simulink model "target_transmit"  (R2018a)
settings: Solver=FixedStepDiscrete  StartTime=0  StopTime=inf  RelTol=1e-3  EnableMultiTasking=on
InitFcn:
  | load data/bestsimulink_data
  | load data/bestsimulink320x240_data
  | load busObjects
StopFcn:
  | clear bestsimulink320x240_data
  | clear bestsimulink_data
  | clear dataBusObject
model workspace (MAT data in the model file):
  dt = 0.1
undefined symbols (not defined in the file or in its folder): gray, IsPositionTracked, IsSkeletonTracked, JointDepthIndices, JointImageIndices, JointTrackingState, JointWorldCoordinates, none, PositionDepthIndices, PositionImageIndices, PositionWorldCoordinates, Rec, SDTV, SegmentationData, SkeletonTrackingID, videoinput
libraries: visiontextngfix x24, embdlinuxlib x13, visionstatistics x7, visionconversions x5, visiontransforms x3, visionsinks x2, visionanalysis x1, dspvision x1, imaqlib x1, sldrtlib x1
(part 2 of 2)

== system target_transmit/Draw Bounding Boxes/No Comparison/Insert Buoy Blobs1 ==
  Video In : Inport
  Blob Data : Inport  Port=2
  Bus Selector : BusSelector  OutputSignals=green_bbox,red_bbox
  Draw Shapes Green : visiontextngfix/Draw Shapes  shape=Rectangles  fill=on  lineWidth=1  fillClrSource=Specify via dialog  display=User-specified value  intensity=200  color=[0 255 0]  opacity=0.6  viewport=Entire image  antialiasing=off  inType=Obsolete  imagePorts=One multidimensional signal  prodOutputMode=Binary point scaling  prodOutputWordLength=32  prodOutputFracLength=14  memoryMode=Specify word length  memoryWordLength=16  memoryFracLength=14  roundingMode=Floor  overflowMode=off
      settings: SourceProductName=Computer Vision System Toolbox
  Draw Shapes Red : visiontextngfix/Draw Shapes  shape=Rectangles  fill=on  lineWidth=1  fillClrSource=Specify via dialog  display=User-specified value  intensity=200  color=[255 0 0]  opacity=0.6  viewport=Entire image  antialiasing=off  inType=Obsolete  imagePorts=One multidimensional signal  prodOutputMode=Binary point scaling  prodOutputWordLength=32  prodOutputFracLength=14  memoryMode=Specify word length  memoryWordLength=16  memoryFracLength=14  roundingMode=Floor  overflowMode=off
      settings: SourceProductName=Computer Vision System Toolbox
  Video Out : Outport
  wires:
  Blob Data/1 -> Bus Selector/1
  Video In/1 -> Draw Shapes Green/1
  Draw Shapes Green/1 -> Draw Shapes Red/1
  Draw Shapes Red/1 -> Video Out/1
  Bus Selector/1 -> Draw Shapes Green/2  "<green_bbox>"
  Bus Selector/2 -> Draw Shapes Red/2  "<red_bbox>"

== system target_transmit/Draw Bounding Boxes/No Comparison/Insert Closest Text ==
  Video In : Inport
  Blob Data : Inport  Port=2
  Bus Selector : BusSelector  OutputSignals=green_area,green_centroid,green_bbox,red_area,red_centroid,red_bbox
  Convert Bus to Double : Subsystem  Commented=on
  Find Closest Buoy : MATLAB Function  TreatAsAtomicUnit=on
  Insert Text Green Closest : visiontextngfix/Insert Text  inputType=Obsolete  theText='Closest Green Buoy'  getTextLocFrom=Input port  textLoc=[1 1]  getTextColorFrom=Specify via dialog  textColor=[0 255 0]  getTextIntensityFrom=Specify via dialog  textIntensity=0  getTextOpacityFrom=Specify via dialog  textOpacity=1.0  dummyVar2=0  dummyVar3=0  dummyVar4=0  imagePorts=One multidimensional signal  isInputTransposed=off  fontFace=LucidaSansRegular  dummyVar1=0  blockFontSize=12  antiAliased=on
      settings: SourceProductName=Computer Vision System Toolbox  SourceProductBaseCode=VP
  Insert Text Red Closest : visiontextngfix/Insert Text  inputType=Obsolete  theText='Closest Red Buoy'  getTextLocFrom=Input port  textLoc=[1 1]  getTextColorFrom=Specify via dialog  textColor=[255 0 0]  getTextIntensityFrom=Specify via dialog  textIntensity=0  getTextOpacityFrom=Specify via dialog  textOpacity=1.0  dummyVar2=0  dummyVar3=0  dummyVar4=0  imagePorts=One multidimensional signal  isInputTransposed=off  fontFace=LucidaSansRegular  dummyVar1=0  blockFontSize=12  antiAliased=on
      settings: SourceProductName=Computer Vision System Toolbox  SourceProductBaseCode=VP
  To Workspace : ToWorkspace  Commented=on  VariableName=data1  SaveFormat=Timeseries  SampleTime=-1
  Video Out : Outport
  wires:
  Insert Text Green Closest/1 -> Insert Text Red Closest/1
  Video In/1 -> Insert Text Green Closest/1
  Insert Text Red Closest/1 -> Video Out/1
  Find Closest Buoy/1(gcoord) -> Insert Text Green Closest/2
  Find Closest Buoy/2(rcoord) -> Insert Text Red Closest/2
  Blob Data/1 -> Bus Selector/1
  Bus Selector/3 -> Find Closest Buoy/3(green_bbox)  "<green_bbox>"
  Bus Selector/4 -> Find Closest Buoy/4(red_area)  "<red_area>"
  Bus Selector/2 -> Find Closest Buoy/2(green_centroid)  "<green_centroid>"
  Bus Selector/5 -> Find Closest Buoy/5(red_centroid)  "<red_centroid>"
  Bus Selector/1 -> Find Closest Buoy/1(green_area)  "<green_area>"
  Bus Selector/6 -> Find Closest Buoy/6(red_bbox)  "<red_bbox>"
  Find Closest Buoy/3(data) -> Convert Bus to Double/1(input)
  Convert Bus to Double/1(output) -> To Workspace/1

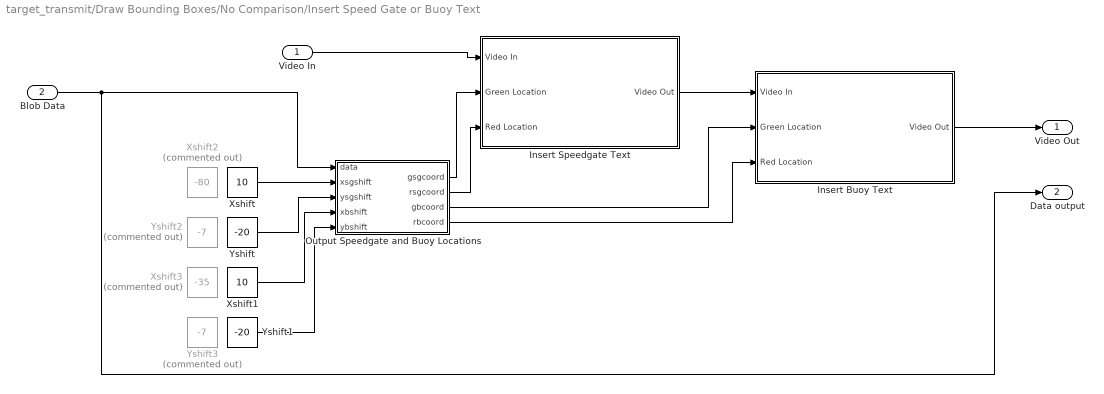
== system target_transmit/Draw Bounding Boxes/No Comparison/Insert Speed Gate or Buoy Text ==
  Video In : Inport
  Blob Data : Inport  Port=2
  Insert Buoy Text : Subsystem
  Insert Speedgate Text : Subsystem
  Output Speedgate and Buoy Locations : MATLAB Function  TreatAsAtomicUnit=on
  Xshift : Constant  Value=10
  Xshift1 : Constant  Value=10
  Xshift2 : Constant  Commented=on  Value=-80
  Xshift3 : Constant  Commented=on  Value=-35
  Yshift : Constant  Value=-20
  Yshift1 : Constant  Value=-20
  Yshift2 : Constant  Commented=on  Value=-7
  Yshift3 : Constant  Commented=on  Value=-7
  Video Out : Outport
  Data output : Outport  Port=2
  wires:
  Video In/1 -> Insert Speedgate Text/1(Video In)
  Insert Speedgate Text/1(Video Out) -> Insert Buoy Text/1(Video In)
  Insert Buoy Text/1(Video Out) -> Video Out/1
  Output Speedgate and Buoy Locations/1(gsgcoord) -> Insert Speedgate Text/2(Green Location)
  Output Speedgate and Buoy Locations/2(rsgcoord) -> Insert Speedgate Text/3(Red Location)
  Output Speedgate and Buoy Locations/3(gbcoord) -> Insert Buoy Text/2(Green Location)
  Output Speedgate and Buoy Locations/4(rbcoord) -> Insert Buoy Text/3(Red Location)
  Xshift/1 -> Output Speedgate and Buoy Locations/2(xsgshift)
  Yshift/1 -> Output Speedgate and Buoy Locations/3(ysgshift)
  Xshift1/1 -> Output Speedgate and Buoy Locations/4(xbshift)
  Yshift1/1 -> Output Speedgate and Buoy Locations/5(ybshift)
  Blob Data/1 -> Data output/1, Output Speedgate and Buoy Locations/1(data)

== system target_transmit/Draw Bounding Boxes/No Comparison/Reflection Removal ==
  Blob Data In : Inport
  Bus Creator : BusCreator  Inputs=6
  Bus Selector2 : BusSelector  OutputSignals=green_area,green_centroid,green_bbox,red_area,red_centroid,red_bbox
  Green Reflection Removal : MATLAB Function  TreatAsAtomicUnit=on
  Red Reflection Removal : MATLAB Function  TreatAsAtomicUnit=on
  Blob Data Out : Outport
  wires:
  Bus Creator/1 -> Blob Data Out/1
  Blob Data In/1 -> Bus Selector2/1
  Bus Selector2/1 -> Green Reflection Removal/1(blob_area_in)  "<green_area>"
  Bus Selector2/2 -> Green Reflection Removal/2(blob_centroid_in)  "<green_centroid>"
  Bus Selector2/3 -> Green Reflection Removal/3(blob_bbox_in)  "<green_bbox>"
  Bus Selector2/5 -> Red Reflection Removal/2(blob_centroid_in)  "<red_centroid>"
  Bus Selector2/6 -> Red Reflection Removal/3(blob_bbox_in)  "<red_bbox>"
  Bus Selector2/4 -> Red Reflection Removal/1(blob_area_in)  "<red_area>"
  Green Reflection Removal/1(blob_area_out) -> Bus Creator/1  "green_area"
  Green Reflection Removal/2(blob_centroid_out) -> Bus Creator/2  "green_centroid"
  Green Reflection Removal/3(blob_bbox_out) -> Bus Creator/3  "green_bbox"
  Red Reflection Removal/2(blob_centroid_out) -> Bus Creator/5  "red_centroid"
  Red Reflection Removal/1(blob_area_out) -> Bus Creator/4  "red_area"
  Red Reflection Removal/3(blob_bbox_out) -> Bus Creator/6  "red_bbox"

== system target_transmit/Draw Bounding Boxes/Comparison/Insert Area Text/Obtain Coordinates for Green Area Labels ==
  Green centroid : Inport
  Green bbox : Inport  Port=2
  Add : Sum
  Bias : Bias  Bias=10
  Bias1 : Bias  Bias=-7
  Data Type Conversion2 : DataTypeConversion
  Selector : Selector  NumberOfDimensions=2  InputPortWidth=3  IndexOptions=Select all,Index vector (dialog)  Indices=[1 3],1  OutputSizes=1,1
  Selector1 : Selector  NumberOfDimensions=2  InputPortWidth=3  IndexOptions=Select all,Index vector (dialog)  Indices=[1 3],2  OutputSizes=1,1
  Selector2 : Selector  NumberOfDimensions=2  InputPortWidth=3  IndexOptions=Select all,Index vector (dialog)  Indices=[1 3],3  OutputSizes=1,1
  Vector Concatenate : Concatenate  Mode=Multidimensional array  ConcatenateDimension=2
  Green Area Coord : Outport
  wires:
  Green centroid/1 -> Selector1/1
  Green bbox/1 -> Selector/1, Selector2/1
  Bias1/1 -> Vector Concatenate/2
  Data Type Conversion2/1 -> Green Area Coord/1
  Bias/1 -> Vector Concatenate/1
  Selector/1 -> Add/1
  Add/1 -> Bias/1  "x bbox right"
  Vector Concatenate/1 -> Data Type Conversion2/1
  Selector2/1 -> Add/2
  Selector1/1 -> Bias1/1  "y centroid"

== system target_transmit/Draw Bounding Boxes/Comparison/Insert Area Text/Obtain Coordinates for Red Area Labels1 ==
  Red centroid : Inport
  Red bbox : Inport  Port=2
  Add : Sum
  Bias : Bias  Bias=10
  Bias1 : Bias  Bias=-7
  Data Type Conversion2 : DataTypeConversion
  Selector : Selector  NumberOfDimensions=2  InputPortWidth=3  IndexOptions=Select all,Index vector (dialog)  Indices=[1 3],1  OutputSizes=1,1
  Selector1 : Selector  NumberOfDimensions=2  InputPortWidth=3  IndexOptions=Select all,Index vector (dialog)  Indices=[1 3],2  OutputSizes=1,1
  Selector2 : Selector  NumberOfDimensions=2  InputPortWidth=3  IndexOptions=Select all,Index vector (dialog)  Indices=[1 3],3  OutputSizes=1,1
  Vector Concatenate : Concatenate  Mode=Multidimensional array  ConcatenateDimension=2
  Red Area Coord : Outport
  wires:
  Selector1/1 -> Bias1/1  "y centroid"
  Selector2/1 -> Add/2
  Vector Concatenate/1 -> Data Type Conversion2/1
  Add/1 -> Bias/1  "x bbox right"
  Selector/1 -> Add/1
  Bias/1 -> Vector Concatenate/1
  Data Type Conversion2/1 -> Red Area Coord/1
  Bias1/1 -> Vector Concatenate/2
  Red bbox/1 -> Selector2/1, Selector/1
  Red centroid/1 -> Selector1/1

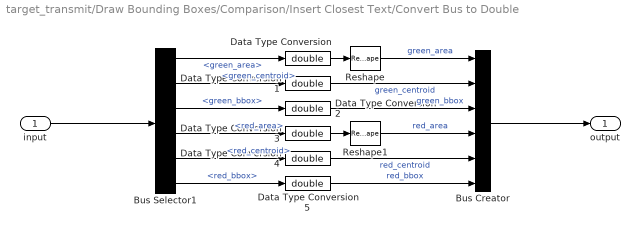
== system target_transmit/Draw Bounding Boxes/Comparison/Insert Closest Text/Convert Bus to Double ==
  input : Inport
  Bus Creator : BusCreator  Inputs=6
  Bus Selector1 : BusSelector  OutputSignals=green_area,green_centroid,green_bbox,red_area,red_centroid,red_bbox
  Data Type Conversion{,1..5} (6 alike) : DataTypeConversion  OutDataTypeStr=double
  Reshape : Reshape
  Reshape1 : Reshape
  output : Outport
  wires:
  Reshape1/1 -> Bus Creator/4  "red_area"
  Reshape/1 -> Bus Creator/1  "green_area"
  Data Type Conversion5/1 -> Bus Creator/6  "red_bbox"
  Data Type Conversion4/1 -> Bus Creator/5  "red_centroid"
  Data Type Conversion3/1 -> Reshape1/1
  Data Type Conversion2/1 -> Bus Creator/3  "green_bbox"
  Data Type Conversion1/1 -> Bus Creator/2  "green_centroid"
  Data Type Conversion/1 -> Reshape/1
  Bus Selector1/1 -> Data Type Conversion/1  "<green_area>"
  Bus Selector1/3 -> Data Type Conversion2/1  "<green_bbox>"
  Bus Selector1/2 -> Data Type Conversion1/1  "<green_centroid>"
  Bus Selector1/5 -> Data Type Conversion4/1  "<red_centroid>"
  Bus Selector1/6 -> Data Type Conversion5/1  "<red_bbox>"
  Bus Selector1/4 -> Data Type Conversion3/1  "<red_area>"
  input/1 -> Bus Selector1/1
  Bus Creator/1 -> output/1

== system target_transmit/Draw Bounding Boxes/Comparison/Insert Speed Gate or Buoy Text/Insert Buoy Text ==
  Video In : Inport
  Green Location : Inport  Port=2
  Red Location : Inport  Port=3
  Data Type Conversion : DataTypeConversion
  Data Type Conversion2 : DataTypeConversion
  Insert Text Green Area : visiontextngfix/Insert Text  inputType=Obsolete  theText='Buoy'  fontFace=LucidaSansRegular  dummyVar1=0  blockFontSize=12  antiAliased=on  getTextLocFrom=Input port  textLoc=[1 1]  getTextColorFrom=Specify via dialog  textColor=[0 255 0]  getTextIntensityFrom=Specify via dialog  textIntensity=0  getTextOpacityFrom=Specify via dialog  textOpacity=1.0  dummyVar2=0  dummyVar3=0  dummyVar4=0  imagePorts=One multidimensional signal  isInputTransposed=off
      settings: SourceProductName=Computer Vision System Toolbox  SourceProductBaseCode=VP
  Insert Text Red Area : visiontextngfix/Insert Text  inputType=Obsolete  theText='Buoy'  fontFace=LucidaSansRegular  dummyVar1=0  blockFontSize=12  antiAliased=on  getTextLocFrom=Input port  textLoc=[1 1]  getTextColorFrom=Specify via dialog  textColor=[255 0 0]  getTextIntensityFrom=Specify via dialog  textIntensity=0  getTextOpacityFrom=Specify via dialog  textOpacity=1.0  dummyVar2=0  dummyVar3=0  dummyVar4=0  imagePorts=One multidimensional signal  isInputTransposed=off
      settings: SourceProductName=Computer Vision System Toolbox  SourceProductBaseCode=VP
  Video Out : Outport
  wires:
  Data Type Conversion2/1 -> Insert Text Red Area/2
  Insert Text Green Area/1 -> Insert Text Red Area/1  "video"
  Data Type Conversion/1 -> Insert Text Green Area/2
  Green Location/1 -> Data Type Conversion/1
  Red Location/1 -> Data Type Conversion2/1
  Video In/1 -> Insert Text Green Area/1
  Insert Text Red Area/1 -> Video Out/1  "video"

== system target_transmit/Draw Bounding Boxes/Comparison/Insert Speed Gate or Buoy Text/Insert Speedgate Text ==
  Video In : Inport
  Green Location : Inport  Port=2
  Red Location : Inport  Port=3
  Data Type Conversion : DataTypeConversion
  Data Type Conversion2 : DataTypeConversion
  Insert Text Green Area : visiontextngfix/Insert Text  inputType=Obsolete  theText='Speed Gate'  fontFace=LucidaSansRegular  dummyVar1=0  blockFontSize=12  antiAliased=on  getTextLocFrom=Input port  textLoc=[1 1]  getTextColorFrom=Specify via dialog  textColor=[0 255 0]  getTextIntensityFrom=Specify via dialog  textIntensity=0  getTextOpacityFrom=Specify via dialog  textOpacity=1.0  dummyVar2=0  dummyVar3=0  dummyVar4=0  imagePorts=One multidimensional signal  isInputTransposed=off
      settings: SourceProductName=Computer Vision System Toolbox  SourceProductBaseCode=VP
  Insert Text Red Area : visiontextngfix/Insert Text  inputType=Obsolete  theText='Speed Gate'  fontFace=LucidaSansRegular  dummyVar1=0  blockFontSize=12  antiAliased=on  getTextLocFrom=Input port  textLoc=[1 1]  getTextColorFrom=Specify via dialog  textColor=[255 0 0]  getTextIntensityFrom=Specify via dialog  textIntensity=0  getTextOpacityFrom=Specify via dialog  textOpacity=1.0  dummyVar2=0  dummyVar3=0  dummyVar4=0  imagePorts=One multidimensional signal  isInputTransposed=off
      settings: SourceProductName=Computer Vision System Toolbox  SourceProductBaseCode=VP
  Video Out : Outport
  wires:
  Insert Text Red Area/1 -> Video Out/1  "video"
  Video In/1 -> Insert Text Green Area/1
  Red Location/1 -> Data Type Conversion2/1
  Green Location/1 -> Data Type Conversion/1
  Data Type Conversion/1 -> Insert Text Green Area/2
  Insert Text Green Area/1 -> Insert Text Red Area/1  "video"
  Data Type Conversion2/1 -> Insert Text Red Area/2

== system target_transmit/Draw Bounding Boxes/No Comparison/Insert Area Text/Obtain Coordinates for Green Area Labels ==
  Green centroid : Inport
  Green bbox : Inport  Port=2
  Add : Sum
  Bias : Bias  Bias=10
  Bias1 : Bias  Bias=-7
  Data Type Conversion2 : DataTypeConversion
  Selector : Selector  NumberOfDimensions=2  InputPortWidth=3  IndexOptions=Select all,Index vector (dialog)  Indices=[1 3],1  OutputSizes=1,1
  Selector1 : Selector  NumberOfDimensions=2  InputPortWidth=3  IndexOptions=Select all,Index vector (dialog)  Indices=[1 3],2  OutputSizes=1,1
  Selector2 : Selector  NumberOfDimensions=2  InputPortWidth=3  IndexOptions=Select all,Index vector (dialog)  Indices=[1 3],3  OutputSizes=1,1
  Vector Concatenate : Concatenate  Mode=Multidimensional array  ConcatenateDimension=2
  Green Area Coord : Outport
  wires:
  Selector1/1 -> Bias1/1  "y centroid"
  Selector2/1 -> Add/2
  Vector Concatenate/1 -> Data Type Conversion2/1
  Add/1 -> Bias/1  "x bbox right"
  Selector/1 -> Add/1
  Bias/1 -> Vector Concatenate/1
  Data Type Conversion2/1 -> Green Area Coord/1
  Bias1/1 -> Vector Concatenate/2
  Green bbox/1 -> Selector2/1, Selector/1
  Green centroid/1 -> Selector1/1

== system target_transmit/Draw Bounding Boxes/No Comparison/Insert Area Text/Obtain Coordinates for Red Area Labels1 ==
  Red centroid : Inport
  Red bbox : Inport  Port=2
  Add : Sum
  Bias : Bias  Bias=10
  Bias1 : Bias  Bias=-7
  Data Type Conversion2 : DataTypeConversion
  Selector : Selector  NumberOfDimensions=2  InputPortWidth=3  IndexOptions=Select all,Index vector (dialog)  Indices=[1 3],1  OutputSizes=1,1
  Selector1 : Selector  NumberOfDimensions=2  InputPortWidth=3  IndexOptions=Select all,Index vector (dialog)  Indices=[1 3],2  OutputSizes=1,1
  Selector2 : Selector  NumberOfDimensions=2  InputPortWidth=3  IndexOptions=Select all,Index vector (dialog)  Indices=[1 3],3  OutputSizes=1,1
  Vector Concatenate : Concatenate  Mode=Multidimensional array  ConcatenateDimension=2
  Red Area Coord : Outport
  wires:
  Red centroid/1 -> Selector1/1
  Red bbox/1 -> Selector/1, Selector2/1
  Bias1/1 -> Vector Concatenate/2
  Data Type Conversion2/1 -> Red Area Coord/1
  Bias/1 -> Vector Concatenate/1
  Selector/1 -> Add/1
  Add/1 -> Bias/1  "x bbox right"
  Vector Concatenate/1 -> Data Type Conversion2/1
  Selector2/1 -> Add/2
  Selector1/1 -> Bias1/1  "y centroid"

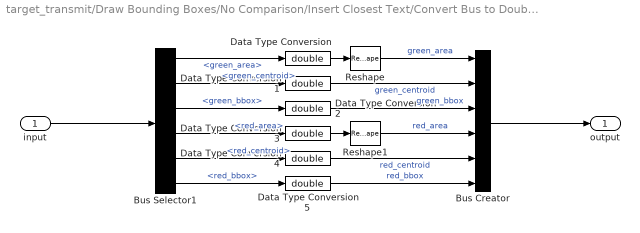
== system target_transmit/Draw Bounding Boxes/No Comparison/Insert Closest Text/Convert Bus to Double ==
  input : Inport
  Bus Creator : BusCreator  Inputs=6
  Bus Selector1 : BusSelector  OutputSignals=green_area,green_centroid,green_bbox,red_area,red_centroid,red_bbox
  Data Type Conversion{,1..5} (6 alike) : DataTypeConversion  OutDataTypeStr=double
  Reshape : Reshape
  Reshape1 : Reshape
  output : Outport
  wires:
  Bus Creator/1 -> output/1
  input/1 -> Bus Selector1/1
  Bus Selector1/4 -> Data Type Conversion3/1  "<red_area>"
  Bus Selector1/6 -> Data Type Conversion5/1  "<red_bbox>"
  Bus Selector1/5 -> Data Type Conversion4/1  "<red_centroid>"
  Bus Selector1/2 -> Data Type Conversion1/1  "<green_centroid>"
  Bus Selector1/3 -> Data Type Conversion2/1  "<green_bbox>"
  Bus Selector1/1 -> Data Type Conversion/1  "<green_area>"
  Data Type Conversion/1 -> Reshape/1
  Data Type Conversion1/1 -> Bus Creator/2  "green_centroid"
  Data Type Conversion2/1 -> Bus Creator/3  "green_bbox"
  Data Type Conversion3/1 -> Reshape1/1
  Data Type Conversion4/1 -> Bus Creator/5  "red_centroid"
  Data Type Conversion5/1 -> Bus Creator/6  "red_bbox"
  Reshape/1 -> Bus Creator/1  "green_area"
  Reshape1/1 -> Bus Creator/4  "red_area"

== system target_transmit/Draw Bounding Boxes/No Comparison/Insert Speed Gate or Buoy Text/Insert Buoy Text ==
  Video In : Inport
  Green Location : Inport  Port=2
  Red Location : Inport  Port=3
  Data Type Conversion : DataTypeConversion
  Data Type Conversion2 : DataTypeConversion
  Insert Text Green Area : visiontextngfix/Insert Text  inputType=Obsolete  theText='Buoy'  fontFace=LucidaSansRegular  dummyVar1=0  blockFontSize=12  antiAliased=on  getTextLocFrom=Input port  textLoc=[1 1]  getTextColorFrom=Specify via dialog  textColor=[0 255 0]  getTextIntensityFrom=Specify via dialog  textIntensity=0  getTextOpacityFrom=Specify via dialog  textOpacity=1.0  dummyVar2=0  dummyVar3=0  dummyVar4=0  imagePorts=One multidimensional signal  isInputTransposed=off
      settings: SourceProductName=Computer Vision System Toolbox  SourceProductBaseCode=VP
  Insert Text Red Area : visiontextngfix/Insert Text  inputType=Obsolete  theText='Buoy'  fontFace=LucidaSansRegular  dummyVar1=0  blockFontSize=12  antiAliased=on  getTextLocFrom=Input port  textLoc=[1 1]  getTextColorFrom=Specify via dialog  textColor=[255 0 0]  getTextIntensityFrom=Specify via dialog  textIntensity=0  getTextOpacityFrom=Specify via dialog  textOpacity=1.0  dummyVar2=0  dummyVar3=0  dummyVar4=0  imagePorts=One multidimensional signal  isInputTransposed=off
      settings: SourceProductName=Computer Vision System Toolbox  SourceProductBaseCode=VP
  Video Out : Outport
  wires:
  Insert Text Red Area/1 -> Video Out/1  "video"
  Video In/1 -> Insert Text Green Area/1
  Red Location/1 -> Data Type Conversion2/1
  Green Location/1 -> Data Type Conversion/1
  Data Type Conversion/1 -> Insert Text Green Area/2
  Insert Text Green Area/1 -> Insert Text Red Area/1  "video"
  Data Type Conversion2/1 -> Insert Text Red Area/2

== system target_transmit/Draw Bounding Boxes/No Comparison/Insert Speed Gate or Buoy Text/Insert Speedgate Text ==
  Video In : Inport
  Green Location : Inport  Port=2
  Red Location : Inport  Port=3
  Data Type Conversion : DataTypeConversion
  Data Type Conversion2 : DataTypeConversion
  Insert Text Green Area : visiontextngfix/Insert Text  inputType=Obsolete  theText='Speed Gate'  fontFace=LucidaSansRegular  dummyVar1=0  blockFontSize=12  antiAliased=on  getTextLocFrom=Input port  textLoc=[1 1]  getTextColorFrom=Specify via dialog  textColor=[0 255 0]  getTextIntensityFrom=Specify via dialog  textIntensity=0  getTextOpacityFrom=Specify via dialog  textOpacity=1.0  dummyVar2=0  dummyVar3=0  dummyVar4=0  imagePorts=One multidimensional signal  isInputTransposed=off
      settings: SourceProductName=Computer Vision System Toolbox  SourceProductBaseCode=VP
  Insert Text Red Area : visiontextngfix/Insert Text  inputType=Obsolete  theText='Speed Gate'  fontFace=LucidaSansRegular  dummyVar1=0  blockFontSize=12  antiAliased=on  getTextLocFrom=Input port  textLoc=[1 1]  getTextColorFrom=Specify via dialog  textColor=[255 0 0]  getTextIntensityFrom=Specify via dialog  textIntensity=0  getTextOpacityFrom=Specify via dialog  textOpacity=1.0  dummyVar2=0  dummyVar3=0  dummyVar4=0  imagePorts=One multidimensional signal  isInputTransposed=off
      settings: SourceProductName=Computer Vision System Toolbox  SourceProductBaseCode=VP
  Video Out : Outport
  wires:
  Data Type Conversion2/1 -> Insert Text Red Area/2
  Insert Text Green Area/1 -> Insert Text Red Area/1  "video"
  Data Type Conversion/1 -> Insert Text Green Area/2
  Green Location/1 -> Data Type Conversion/1
  Red Location/1 -> Data Type Conversion2/1
  Video In/1 -> Insert Text Green Area/1
  Insert Text Red Area/1 -> Video Out/1  "video"

== matlab function target_transmit/Buoy Detection Algorithm/variant1: Subtraction Based Thresholding 4 Blobs/MATLAB Function1 ==
  data: theta1 input; rho1 input; theta2 input; rho2 input
function fcn(theta1,rho1, theta2, rho2)
    plot(rho1,theta1, 'x')
    plot(rho2,theta2, 'o')

end

== matlab function target_transmit/Buoy Detection Algorithm/variant1: Subtraction Based Thresholding 4 Blobs/MATLAB Function2 ==
  data: theta input; theta_vec output; rho_vec output; rho input
function [theta_vec,rho_vec] = fcn(theta, rho)
    mat =[transpose(theta),transpose(rho)]
    [res,C] = kmeans(mat,3);
    theta
    rho
    C
    theta_vec = transpose([C(:,1)])
    rho_vec = transpose([C(:,2)])
    
    
    
    
%     disp(theta_vec)
%     disp(rho_vec)
%     
%     goalpost_theta = [0];
%     goalpost_rho = [0];
%     res_rho = zeros(1,6);
%     res_theta = zeros(1,6);
%     
%     for i=1:length(theta_vec)
%         if (theta_vec(i) >= 0 && theta_vec(i) < 30)
%             res_theta(i) = theta_vec(i)
%             res_rho(i) = rho_vec(i)
%         end 
%     end
%     
%     disp(goalpost_theta)
%     disp(goalpost_rho)
%     
%     for i=1:length(goalpost_rho)
%         if (goalpost_rho(i) == 0)
%             goalpost_rho(i) = []
%         end
%         if (goalpost_theta(i)  == 0)
%             goalpost_theta(i) = []
%         end
%     end
    
end

== matlab function target_transmit/Draw Bounding Boxes/No Comparison/Reflection Removal/Green Reflection Removal ==
  data: blob_area_in input; blob_centroid_in input; blob_bbox_in input; blob_area_out output; blob_centroid_out output; blob_bbox_out output
function [blob_area_out, blob_centroid_out, blob_bbox_out] = fcn(blob_area_in,blob_centroid_in, blob_bbox_in)
%#codegen
%% buoy reflection removal 

% extract valid blob data
blobidx = find(blob_centroid_in(:,1)~=-1); % locations in original vector where blob data is
nblobs = length(blobidx);

blob_area = blob_area_in(blobidx,:);
blob_centroid = double(blob_centroid_in(blobidx,:)); 
blob_bbox = blob_bbox_in(blobidx,:);

% only perform blob reflection removal if there are more than 1 blobs
if nblobs >=2
    tolXC = 80;
    connectivity = zeros(1,2);
    diffXC = zeros(1,2);

    % create difference and connectivity matrix
    % diffXC = absolute difference between X coordinates of centroids
    % connectivity matrix provides all of the comparisons that can be performed
    if nblobs == 2
        diffXC = abs(blob_centroid(1,1)-blob_centroid(2,1));
        connectivity = [1 2];  
    elseif nblobs == 3
        diffXC = abs([blob_centroid(1,1)-blob_centroid(2,1);
                        blob_centroid(1,1)-blob_centroid(3,1);
                        blob_centroid(2,1)-blob_centroid(3,1)]);
        connectivity = [1 2; 1 3; 2 3];
    elseif nblobs == 4
        diffXC = abs([blob_centroid(1,1)-blob_centroid(2,1);
                        blob_centroid(1,1)-blob_centroid(3,1);
                        blob_centroid(1,1)-blob_centroid(4,1);
                        blob_centroid(2,1)-blob_centroid(3,1);
                        blob_centroid(2,1)-blob_centroid(4,1);
                        blob_centroid(3,1)-blob_centroid(4,1)]);
        connectivity = [1 2; 1 3; 1 4; 2 3; 2 4; 3 4];
    end

    % loop through connectivity matrix to find reflection blobs and remove
    boolXC = diffXC<tolXC;
    for idx = 1:size(connectivity,1);
        if boolXC(idx)
           % remove lower blob corresponding to connectivity(idx,:)
           % find lower blob
           refidx = connectivity(idx,:); % i.e. [1 2] buoys which are possibly reflections

           [~,maxidx] = max(blob_centroid(refidx,2)); % i.e. [2] % buoy which is lowest aka reflection
           [~,minidx] = min(blob_centroid(refidx,2)); 
           
           if blob_area(refidx(maxidx))<blob_area(refidx(minidx)) % if lowest blob's area is smaller than upper blob, remove
               % erase blob data corresponding to reflections
               blob_area(blobidx(refidx(maxidx)),:) = -1;
               blob_centroid(blobidx(refidx(maxidx)),:) = -1;
               blob_bbox(blobidx(refidx(maxidx)),:) = -1;
           end
           % blobidx(refidx) = [2 3];
           % blobidx(refidx(maxidx) = 2;
        end
    end  
end % end of blob removal

% color specific 
% output red data
blob_area_out = -ones(4,1);
blob_centroid_out = -ones(4,2);
blob_bbox_out = -ones(4,4);

blob_area_out(1:nblobs) = blob_area;
blob_centroid_out(1:nblobs,:) = blob_centroid;
blob_bbox_out(1:nblobs,:) = blob_bbox;

== matlab function target_transmit/Draw Bounding Boxes/No Comparison/Reflection Removal/Red Reflection Removal ==
  data: blob_area_in input; blob_centroid_in input; blob_bbox_in input; blob_area_out output; blob_centroid_out output; blob_bbox_out output
function [blob_area_out, blob_centroid_out, blob_bbox_out] = fcn(blob_area_in,blob_centroid_in, blob_bbox_in)
%#codegen
%% buoy reflection removal 

% extract valid blob data
blobidx = find(blob_centroid_in(:,1)~=-1); % locations in original vector where blob data is
nblobs = length(blobidx);

blob_area = blob_area_in(blobidx,:);
blob_centroid = double(blob_centroid_in(blobidx,:)); 
blob_bbox = blob_bbox_in(blobidx,:);

% only perform blob reflection removal if there are more than 1 blobs
if nblobs >=2
    tolXC = 20;
    connectivity = zeros(1,2);
    diffXC = zeros(1,2);

    % create difference and connectivity matrix
    % diffXC = absolute difference between X coordinates of centroids
    % connectivity matrix provides all of the comparisons that can be performed
    if nblobs == 2
        diffXC = abs(blob_centroid(1,1)-blob_centroid(2,1));
        connectivity = [1 2];  
    elseif nblobs == 3
        diffXC = abs([blob_centroid(1,1)-blob_centroid(2,1);
                        blob_centroid(1,1)-blob_centroid(3,1);
                        blob_centroid(2,1)-blob_centroid(3,1)]);
        connectivity = [1 2; 1 3; 2 3];
    elseif nblobs == 4
        diffXC = abs([blob_centroid(1,1)-blob_centroid(2,1);
                        blob_centroid(1,1)-blob_centroid(3,1);
                        blob_centroid(1,1)-blob_centroid(4,1);
                        blob_centroid(2,1)-blob_centroid(3,1);
                        blob_centroid(2,1)-blob_centroid(4,1);
                        blob_centroid(3,1)-blob_centroid(4,1)]);
        connectivity = [1 2; 1 3; 1 4; 2 3; 2 4; 3 4];
    end

    % loop through connectivity matrix to find reflection blobs and remove
    boolXC = diffXC<tolXC;
    for idx = 1:size(connectivity,1);
        if boolXC(idx)
           % remove lower blob corresponding to connectivity(idx,:)
           % find lower blob
           refidx = connectivity(idx,:); % i.e. [1 2] buoys which are possibly reflections

           [~,maxidx] = max(blob_centroid(refidx,2)); % i.e. [2] % buoy which is lowest aka reflection
           [~,minidx] = min(blob_centroid(refidx,2)); 
           
           if blob_area(refidx(maxidx))<blob_area(refidx(minidx)) % if lowest blob's area is smaller than upper blob, remove
               % erase blob data corresponding to reflections
               blob_area(blobidx(refidx(maxidx)),:) = -1;
               blob_centroid(blobidx(refidx(maxidx)),:) = -1;
               blob_bbox(blobidx(refidx(maxidx)),:) = -1;
           end
           % blobidx(refidx) = [2 3];
           % blobidx(refidx(maxidx) = 2;
        end
    end  
end % end of blob removal

% color specific 
% output red data
blob_area_out = -ones(4,1);
blob_centroid_out = -ones(4,2);
blob_bbox_out = -ones(4,4);

blob_area_out(1:nblobs) = blob_area;
blob_centroid_out(1:nblobs,:) = blob_centroid;
blob_bbox_out(1:nblobs,:) = blob_bbox;

== matlab function target_transmit/Draw Bounding Boxes/Comparison/Insert Closest Text/Find Closest Buoy ==
  data: green_area input; green_centroid input; gcoord output; green_bbox input; red_area input; red_centroid input; red_bbox input; rcoord output; data output Bus: dataBusObject
function [gcoord, rcoord,data] = fcn(green_area,green_centroid,green_bbox,red_area,red_centroid,red_bbox)
%#codegen

% store idx as a persistent variable
persistent idx
if isempty(idx)
   idx = -1; 
end

%% increment the idx of the simulation
idx = idx + 1;

%% identify and remove buoys from the other track
trackID = 1; % 1 == left track, 2 == right track
if trackID==1
    % if boat is on left track remove red buoys to the right of the green speed gates
    % determine which blob is a speed gate
    gh = green_bbox(:,4);
    gw = green_bbox(:,3);
    % gsgidx = Green Speed Gate Idx, points to the buoys which are green
    % speed gates
    gsgidx = find(green_area>100 & gh./gw>3);
    if ~isempty(gsgidx)
        % gr is the coordiante of the right side of the green buoys
        gr = green_bbox(gsgidx(1),1)+green_bbox(gsgidx(1),3);
        % find red buoys that are on the second track and remove them
        rl = red_bbox(:,1);
        rstidx = find(rl>gr); 
        red_area(rstidx) = -1;
        red_centroid(rstidx,:) = -1;
        red_bbox(rstidx,:) = -1;
    end
elseif trackID==2
    % if boat is on the right track, remove green buoys to the left of the red speed gates
        % if boat is on left track remove red buoys to the right of the green speed gates
    % determine which blob is a speed gate
    rh = red_bbox(:,4);
    rw = red_bbox(:,3);
    rsgidx = find(red_area>100 & rh./rw>3);
    if ~isempty(rsgidx)
        % rl is the coordinate of the left side of the red buoys
        rl = red_bbox(rsgidx(1),1);
        % find red buoys that are on the second track and remove them
        gr = green_bbox(:,1)+green_bbox(:,3);
        gstidx = find(gr<rl); 
        green_area(gstidx) = -1;
        green_centroid(gstidx,:) = -1;
        green_bbox(gstidx,:) = -1;
    end
end

%% remove buoys from certain frames that are known to not be in the correct lane
badIdx_green = [812:823 855:875]; % frames are manually chosen
badIdx_red = [785:829 848:879 1276:1285]; % frames are manually chosen
boolBad_green = find(idx == badIdx_green);
boolBad_red = find(idx == badIdx_red);

if ~isempty(boolBad_green)
    green_area = -ones(4,1);
    green_centroid = -ones(4,2);
    green_bbox = -ones(4,4);
end

if ~isempty(boolBad_red)
    red_area = -ones(4,1);
    red_centroid = -ones(4,2);
    red_bbox = -ones(4,4);
end

%% store data into a bus
data.green_area = green_area;
data.green_centroid = green_centroid;
data.green_bbox = green_bbox;
data.red_area = red_area;
data.red_centroid = red_centroid;
data.red_bbox = red_bbox;

%% return coordinates for the closest buoy text
[~, green_closestBuoyIdx] = max(green_bbox(:,2)+green_bbox(:,4));
gcoord = int16([green_centroid(green_closestBuoyIdx,1)-20 green_bbox(green_closestBuoyIdx,2)-15]);

[~, red_closestBuoyIdx] = max(red_bbox(:,2)+red_bbox(:,4));
rcoord = int16([red_centroid(red_closestBuoyIdx,1)-20 red_bbox(red_closestBuoyIdx,2)-15]);

== matlab function target_transmit/Draw Bounding Boxes/Comparison/Insert Speed Gate or Buoy Text/Output Speedgate and Buoy Locations ==
  data: data input Bus: dataBusObject; gsgcoord output size=[4 2]; rsgcoord output size=[4 2]; xsgshift input; ysgshift input; gbcoord output size=[4 2]; rbcoord output size=[4 2]; xbshift input; ybshift input
function [gsgcoord,rsgcoord,gbcoord,rbcoord]= fcn(data,xsgshift,ysgshift,xbshift,ybshift)
%#codegen
    % define thresholds
    athreshold = 500;
    hwthreshold = 25;

    % determine which green blob is a speed gate
    gh = data.green_bbox(:,4);
    gw = data.green_bbox(:,3);
    % gsgidx = Green Speed Gate Idx, points to the buoys which are green
    % speed gates
    
    gsgidx = find(data.green_area>athreshold & gh-gw>hwthreshold);
    gsgcoord = [data.green_bbox(gsgidx,1)+gw(gsgidx)+xsgshift data.green_centroid(gsgidx,2)+ysgshift];
    gbidx = find(gh-gw<hwthreshold);
    gbcoord = [data.green_bbox(gbidx,1)+gw(gbidx)+xbshift data.green_centroid(gbidx,2)+ybshift];
    
    % determine which red blob is a speed gate
    rh = data.red_bbox(:,4);
    rw = data.red_bbox(:,3);
    % gsgidx = red Speed Gate Idx, points to the buoys which are red
    % speed gates
    rsgidx = find(data.red_area>athreshold & rh-rw>hwthreshold);
    rsgcoord = [data.red_bbox(rsgidx,1)+rw(rsgidx)+xsgshift data.red_centroid(rsgidx,2)+ysgshift];
    rbidx = find(rh-rw<hwthreshold);
    rbcoord = [data.red_bbox(rbidx,1)++rw(rbidx)+xbshift data.red_centroid(rbidx,2)+ybshift];

== matlab function target_transmit/Draw Bounding Boxes/No Comparison/Insert Closest Text/Find Closest Buoy ==
  data: green_area input; green_centroid input; gcoord output; green_bbox input; red_area input; red_centroid input; red_bbox input; rcoord output; data output Bus: dataBusObject
function [gcoord, rcoord,data] = fcn(green_area,green_centroid,green_bbox,red_area,red_centroid,red_bbox)
%#codegen

% store idx as a persistent variable
persistent idx
if isempty(idx)
   idx = -1; 
end

%% increment the idx of the simulation
idx = idx + 1;

%% identify and remove buoys from the other track
trackID = 1; % 1 == left track, 2 == right track
if trackID==1
    % if boat is on left track remove red buoys to the right of the green speed gates
    % determine which blob is a speed gate
    gh = green_bbox(:,4);
    gw = green_bbox(:,3);
    % gsgidx = Green Speed Gate Idx, points to the buoys which are green
    % speed gates
    gsgidx = find(green_area>100 & gh./gw>3);
    if ~isempty(gsgidx)
        % gr is the coordiante of the right side of the green buoys
        gr = green_bbox(gsgidx(1),1)+green_bbox(gsgidx(1),3);
        % find red buoys that are on the second track and remove them
        rl = red_bbox(:,1);
        rstidx = find(rl>gr); 
        red_area(rstidx) = -1;
        red_centroid(rstidx,:) = -1;
        red_bbox(rstidx,:) = -1;
    end
elseif trackID==2
    % if boat is on the right track, remove green buoys to the left of the red speed gates
        % if boat is on left track remove red buoys to the right of the green speed gates
    % determine which blob is a speed gate
    rh = red_bbox(:,4);
    rw = red_bbox(:,3);
    rsgidx = find(red_area>100 & rh./rw>3);
    if ~isempty(rsgidx)
        % rl is the coordinate of the left side of the red buoys
        rl = red_bbox(rsgidx(1),1);
        % find red buoys that are on the second track and remove them
        gr = green_bbox(:,1)+green_bbox(:,3);
        gstidx = find(gr<rl); 
        green_area(gstidx) = -1;
        green_centroid(gstidx,:) = -1;
        green_bbox(gstidx,:) = -1;
    end
end

%% remove buoys from certain frames that are known to not be in the correct lane
badIdx_green = [812:823 855:875]; % frames are manually chosen
badIdx_red = [785:829 848:879 1276:1285]; % frames are manually chosen
boolBad_green = find(idx == badIdx_green);
boolBad_red = find(idx == badIdx_red);

if ~isempty(boolBad_green)
    green_area = -ones(4,1);
    green_centroid = -ones(4,2);
    green_bbox = -ones(4,4);
end

if ~isempty(boolBad_red)
    red_area = -ones(4,1);
    red_centroid = -ones(4,2);
    red_bbox = -ones(4,4);
end

%% store data into a bus
data.green_area = green_area;
data.green_centroid = green_centroid;
data.green_bbox = green_bbox;
data.red_area = red_area;
data.red_centroid = red_centroid;
data.red_bbox = red_bbox;

%% return coordinates for the closest buoy text
[~, green_closestBuoyIdx] = max(green_bbox(:,2)+green_bbox(:,4));
gcoord = int16([green_centroid(green_closestBuoyIdx,1)-20 green_bbox(green_closestBuoyIdx,2)-15]);

[~, red_closestBuoyIdx] = max(red_bbox(:,2)+red_bbox(:,4));
rcoord = int16([red_centroid(red_closestBuoyIdx,1)-20 red_bbox(red_closestBuoyIdx,2)-15]);

== matlab function target_transmit/Draw Bounding Boxes/No Comparison/Insert Speed Gate or Buoy Text/Output Speedgate and Buoy Locations ==
  data: data input Bus: dataBusObject; gsgcoord output size=[4 2]; rsgcoord output size=[4 2]; xsgshift input; ysgshift input; gbcoord output size=[4 2]; rbcoord output size=[4 2]; xbshift input; ybshift input
function [gsgcoord,rsgcoord,gbcoord,rbcoord]= fcn(data,xsgshift,ysgshift,xbshift,ybshift)
%#codegen
    % define thresholds
    athreshold = 500;
    hwthreshold = 25;

    % determine which green blob is a speed gate
    gh = data.green_bbox(:,4);
    gw = data.green_bbox(:,3);
    % gsgidx = Green Speed Gate Idx, points to the buoys which are green
    % speed gates
    
    gsgidx = find(data.green_area>athreshold & gh-gw>hwthreshold);
    gsgcoord = [data.green_bbox(gsgidx,1)+gw(gsgidx)+xsgshift data.green_centroid(gsgidx,2)+ysgshift];
    gbidx = find(gh-gw<hwthreshold);
    gbcoord = [data.green_bbox(gbidx,1)+gw(gbidx)+xbshift data.green_centroid(gbidx,2)+ybshift];
    
    % determine which red blob is a speed gate
    rh = data.red_bbox(:,4);
    rw = data.red_bbox(:,3);
    % gsgidx = red Speed Gate Idx, points to the buoys which are red
    % speed gates
    rsgidx = find(data.red_area>athreshold & rh-rw>hwthreshold);
    rsgcoord = [data.red_bbox(rsgidx,1)+rw(rsgidx)+xsgshift data.red_centroid(rsgidx,2)+ysgshift];
    rbidx = find(rh-rw<hwthreshold);
    rbcoord = [data.red_bbox(rbidx,1)++rw(rbidx)+xbshift data.red_centroid(rbidx,2)+ybshift];

== matlab function target_transmit/Draw Bounding Boxes/Comparison/Reflection Removal/Green Reflection Removal ==
  data: blob_area_in input; blob_centroid_in input; blob_bbox_in input; blob_area_out output; blob_centroid_out output; blob_bbox_out output
function [blob_area_out, blob_centroid_out, blob_bbox_out] = fcn(blob_area_in,blob_centroid_in, blob_bbox_in)
%#codegen
%% buoy reflection removal 

% extract valid blob data
blobidx = find(blob_centroid_in(:,1)~=-1); % locations in original vector where blob data is
nblobs = length(blobidx);

blob_area = blob_area_in(blobidx,:);
blob_centroid = double(blob_centroid_in(blobidx,:)); 
blob_bbox = blob_bbox_in(blobidx,:);

% only perform blob reflection removal if there are more than 1 blobs
if nblobs >=2
    tolXC = 80;
    connectivity = zeros(1,2);
    diffXC = zeros(1,2);

    % create difference and connectivity matrix
    % diffXC = absolute difference between X coordinates of centroids
    % connectivity matrix provides all of the comparisons that can be performed
    if nblobs == 2
        diffXC = abs(blob_centroid(1,1)-blob_centroid(2,1));
        connectivity = [1 2];  
    elseif nblobs == 3
        diffXC = abs([blob_centroid(1,1)-blob_centroid(2,1);
                        blob_centroid(1,1)-blob_centroid(3,1);
                        blob_centroid(2,1)-blob_centroid(3,1)]);
        connectivity = [1 2; 1 3; 2 3];
    elseif nblobs == 4
        diffXC = abs([blob_centroid(1,1)-blob_centroid(2,1);
                        blob_centroid(1,1)-blob_centroid(3,1);
                        blob_centroid(1,1)-blob_centroid(4,1);
                        blob_centroid(2,1)-blob_centroid(3,1);
                        blob_centroid(2,1)-blob_centroid(4,1);
                        blob_centroid(3,1)-blob_centroid(4,1)]);
        connectivity = [1 2; 1 3; 1 4; 2 3; 2 4; 3 4];
    end

    % loop through connectivity matrix to find reflection blobs and remove
    boolXC = diffXC<tolXC;
    for idx = 1:size(connectivity,1);
        if boolXC(idx)
           % remove lower blob corresponding to connectivity(idx,:)
           % find lower blob
           refidx = connectivity(idx,:); % i.e. [1 2] buoys which are possibly reflections

           [~,maxidx] = max(blob_centroid(refidx,2)); % i.e. [2] % buoy which is lowest aka reflection
           [~,minidx] = min(blob_centroid(refidx,2)); 
           
           if blob_area(refidx(maxidx))<blob_area(refidx(minidx)) % if lowest blob's area is smaller than upper blob, remove
               % erase blob data corresponding to reflections
               blob_area(blobidx(refidx(maxidx)),:) = -1;
               blob_centroid(blobidx(refidx(maxidx)),:) = -1;
               blob_bbox(blobidx(refidx(maxidx)),:) = -1;
           end
           % blobidx(refidx) = [2 3];
           % blobidx(refidx(maxidx) = 2;
        end
    end  
end % end of blob removal

% color specific 
% output red data
blob_area_out = -ones(4,1);
blob_centroid_out = -ones(4,2);
blob_bbox_out = -ones(4,4);

blob_area_out(1:nblobs) = blob_area;
blob_centroid_out(1:nblobs,:) = blob_centroid;
blob_bbox_out(1:nblobs,:) = blob_bbox;

== matlab function target_transmit/Draw Bounding Boxes/Comparison/Reflection Removal/Red Reflection Removal ==
  data: blob_area_in input; blob_centroid_in input; blob_bbox_in input; blob_area_out output; blob_centroid_out output; blob_bbox_out output
function [blob_area_out, blob_centroid_out, blob_bbox_out] = fcn(blob_area_in,blob_centroid_in, blob_bbox_in)
%#codegen
%% buoy reflection removal 

% extract valid blob data
blobidx = find(blob_centroid_in(:,1)~=-1); % locations in original vector where blob data is
nblobs = length(blobidx);

blob_area = blob_area_in(blobidx,:);
blob_centroid = double(blob_centroid_in(blobidx,:)); 
blob_bbox = blob_bbox_in(blobidx,:);

% only perform blob reflection removal if there are more than 1 blobs
if nblobs >=2
    tolXC = 20;
    connectivity = zeros(1,2);
    diffXC = zeros(1,2);

    % create difference and connectivity matrix
    % diffXC = absolute difference between X coordinates of centroids
    % connectivity matrix provides all of the comparisons that can be performed
    if nblobs == 2
        diffXC = abs(blob_centroid(1,1)-blob_centroid(2,1));
        connectivity = [1 2];  
    elseif nblobs == 3
        diffXC = abs([blob_centroid(1,1)-blob_centroid(2,1);
                        blob_centroid(1,1)-blob_centroid(3,1);
                        blob_centroid(2,1)-blob_centroid(3,1)]);
        connectivity = [1 2; 1 3; 2 3];
    elseif nblobs == 4
        diffXC = abs([blob_centroid(1,1)-blob_centroid(2,1);
                        blob_centroid(1,1)-blob_centroid(3,1);
                        blob_centroid(1,1)-blob_centroid(4,1);
                        blob_centroid(2,1)-blob_centroid(3,1);
                        blob_centroid(2,1)-blob_centroid(4,1);
                        blob_centroid(3,1)-blob_centroid(4,1)]);
        connectivity = [1 2; 1 3; 1 4; 2 3; 2 4; 3 4];
    end

    % loop through connectivity matrix to find reflection blobs and remove
    boolXC = diffXC<tolXC;
    for idx = 1:size(connectivity,1);
        if boolXC(idx)
           % remove lower blob corresponding to connectivity(idx,:)
           % find lower blob
           refidx = connectivity(idx,:); % i.e. [1 2] buoys which are possibly reflections

           [~,maxidx] = max(blob_centroid(refidx,2)); % i.e. [2] % buoy which is lowest aka reflection
           [~,minidx] = min(blob_centroid(refidx,2)); 
           
           if blob_area(refidx(maxidx))<blob_area(refidx(minidx)) % if lowest blob's area is smaller than upper blob, remove
               % erase blob data corresponding to reflections
               blob_area(blobidx(refidx(maxidx)),:) = -1;
               blob_centroid(blobidx(refidx(maxidx)),:) = -1;
               blob_bbox(blobidx(refidx(maxidx)),:) = -1;
           end
           % blobidx(refidx) = [2 3];
           % blobidx(refidx(maxidx) = 2;
        end
    end  
end % end of blob removal

% color specific 
% output red data
blob_area_out = -ones(4,1);
blob_centroid_out = -ones(4,2);
blob_bbox_out = -ones(4,4);

blob_area_out(1:nblobs) = blob_area;
blob_centroid_out(1:nblobs,:) = blob_centroid;
blob_bbox_out(1:nblobs,:) = blob_bbox;
